simulink model "parallelizationTest"  (R2017a)
settings: Solver=FixedStepAuto  StartTime=0.0  StopTime=1  FixedStep=0.1  RelTol=1e-3
settings Model: Creator=TSu  LastModifiedBy=TSu
settings SolverCC: AutoInsertRateTranBlk=on

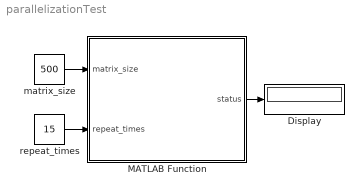
== system parallelizationTest ==
  Display : Display
      settings: Decimation=2
  MATLAB Function : MATLAB Function  TreatAsAtomicUnit=on
  matrix_size : Constant  Value=500
  repeat_times : Constant  Value=15
  wires:
  matrix_size/1 -> MATLAB Function/1(matrix_size)
  repeat_times/1 -> MATLAB Function/2(repeat_times)
  MATLAB Function/1(status) -> Display/1

== matlab function parallelizationTest/MATLAB Function ==
  data: matrix_size input; status output; repeat_times input
function status = time_par_tests(matrix_size, repeat_times)
% time_par_tests: Perform a parallization test (baseline)

status = time_par_tests_mfile(matrix_size, repeat_times);

end
